simulink model "sensorExpoler_lab_Encoder"  (R2026a)
settings: Solver=FixedStepAuto  StopTime=inf  FixedStep=0.001
libraries: simulink x2, amg_usbconverter_n_connect_lib x2, dspfdesign x1
settings Model: Creator=pboon  LastModifiedBy=User

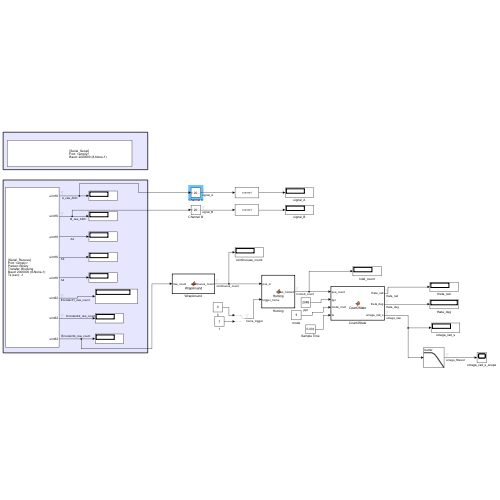
[thumbnail: Simulink's stored preview of the top-level diagram]
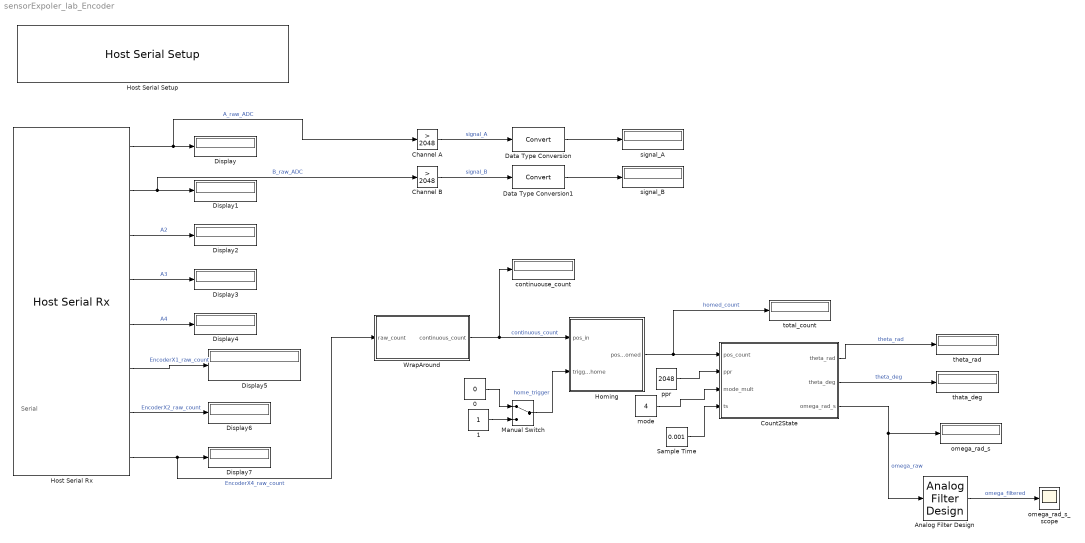
== system sensorExpoler_lab_Encoder ==
  note: Serial
  0 : Constant  Value=0
  1 : Constant
  Analog Filter Design : dspfdesign/Analog Filter Design  method=Butterworth  filttype=Lowpass  N=2  Wlo=30  Whi=80  Rp=2  Rs=40
  Channel A : simulink/Logic and Bit Operations/Compare To Constant  relop=>  const=2048  OutDataTypeStr=boolean
  Channel B : simulink/Logic and Bit Operations/Compare To Constant  relop=>  const=2048  OutDataTypeStr=boolean
  Count2State : MATLAB Function  TreatAsAtomicUnit=on
  Data Type Conversion : DataTypeConversion  SaturateOnIntegerOverflow=off  RndMeth=Floor
  Data Type Conversion1 : DataTypeConversion  SaturateOnIntegerOverflow=off  RndMeth=Floor
  Display{,1..7} (8 alike) : Display
  Homing : MATLAB Function  TreatAsAtomicUnit=on
  Host Serial Rx : amg_usbconverter_n_connect_lib/Host Serial Rx  conf=rx  port=<auto>  baudrate=2000000  databits=8  parity=None  stopbit=1  flowcontrol=None  transfer=Blocking  timeout=5  packetmode=Binary  enableinitialvalues=off  initialvalues=[]  binheader='25'  binterminator='4E 4E'  porttype_double=0  porttype_single=0  porttype_int8=0  porttype_uint8=0  porttype_int16=0  porttype_uint16=5  porttype_int32=0  porttype_uint32=3  asciiformat='%d,%f'  rx_asciiterminator="CRLF (0x0D 0x0A - \"\\r\\n\")"  tx_asciiterminator="CRLF (0x0D 0x0A - \"\\r\\n\")"  sampletime=0.001  enablecustomportlabel=off  cinputportlabel=0  coutputportlabel=A  portpinstr=0  blockid=HostSerialRx  inputporttype=[]  inputportwidth=[]  inputportlabel={}  outputporttype=[5 5 5 5 5 7 7 7]  outputportwidth=[1 1 1 1 1 1 1 1]  outputportlabel={'uint16','uint16','uint16','uint16','uint16','uint32','uint32','uint32'}  compat=0  optionstring=[]  autoport='<empty>'
  Host Serial Setup : amg_usbconverter_n_connect_lib/Host Serial Setup  conf=setup  port=<auto>  baudrate=2000000  databits=8  parity=None  stopbit=1  flowcontrol=None  transfer=Blocking  timeout=2  packetmode=Binary  initialvalues=[]  binheader='7E 7E'  binterminator='03 03'  porttype_double=0  porttype_single=1  porttype_int8=0  porttype_uint8=0  porttype_int16=0  porttype_uint16=0  porttype_int32=0  porttype_uint32=2  asciiformat='%d %u %x'  rx_asciiterminator="CRLF (0x0D 0x0A - \"\\r\\n\")"  tx_asciiterminator="CRLF (0x0D 0x0A - \"\\r\\n\")"  sampletime=-1  enablecustomportlabel=off  cinputportlabel=0  coutputportlabel=A  portpinstr=0  blockid=HostSerialSetup  inputporttype=[]  inputportwidth=[]  inputportlabel={}  outputporttype=[]  outputportwidth=[]  outputportlabel={}  compat=0  optionstring=[]  autoport='<empty>'
  Manual Switch : ManualSwitch
  Sample Time : Constant  Value=0.001
  WrapAround : MATLAB Function  TreatAsAtomicUnit=on
  continuouse_count : Display
  mode : Constant  Value=4
  omega_rad_s : Display
  omega_rad_s_scope : Scope
      settings: ActiveDisplayYMinimum=-168.77272661453941  ActiveDisplayYMaximum=441.86946444637664
  ppr : Constant  Value=2048
  signal_A : Display
  signal_B : Display
  thata_deg : Display
  theta_rad : Display
  total_count : Display
  wires:
  Host Serial Rx/1 -> Channel A/1, Display/1  "A_raw_ADC"
  Host Serial Rx/2 -> Channel B/1, Display1/1  "B_raw_ADC"
  Host Serial Rx/3 -> Display2/1  "A2"
  Host Serial Rx/4 -> Display3/1  "A3"
  Host Serial Rx/7 -> Display6/1  "EncoderX2_raw_count"
  Host Serial Rx/8 -> WrapAround/1(raw_count), Display7/1  "EncoderX4_raw_count"
  Manual Switch/1 -> Homing/2(trigger_home)  "home_trigger"
  ppr/1 -> Count2State/2(ppr)
  mode/1 -> Count2State/3(mode_mult)
  Sample Time/1 -> Count2State/4(ts)
  WrapAround/1(continuous_count) -> continuouse_count/1, Homing/1(pos_in)  "continuous_count"
  1/1 -> Manual Switch/2
  0/1 -> Manual Switch/1
  Count2State/1(theta_rad) -> theta_rad/1  "theta_rad"
  Count2State/2(theta_deg) -> thata_deg/1  "theta_deg"
  Count2State/3(omega_rad_s) -> Analog Filter Design/1, omega_rad_s/1  "omega_raw"
  Host Serial Rx/5 -> Display4/1  "A4"
  Host Serial Rx/6 -> Display5/1  "EncoderX1_raw_count"
  Homing/1(pos_homed) -> total_count/1, Count2State/1(pos_count)  "homed_count"
  Analog Filter Design/1 -> omega_rad_s_scope/1  "omega_filtered"
  Channel A/1 -> Data Type Conversion/1  "signal_A"
  Channel B/1 -> Data Type Conversion1/1  "signal_B"
  Data Type Conversion/1 -> signal_A/1
  Data Type Conversion1/1 -> signal_B/1

== matlab function sensorExpoler_lab_Encoder/Count2State ==
  data: pos_count input; theta_rad output; ppr input; mode_mult input; ts input; theta_deg output; omega_rad_s output
function [theta_rad, theta_deg, omega_rad_s] = Count2State(pos_count, ppr, mode_mult, ts)
    counts_per_rev = double(ppr) * double(mode_mult);
    
    % คำนวณตำแหน่งเชิงมุม
    theta_rad = (double(pos_count) / counts_per_rev) * (2 * pi);
    theta_deg = (double(pos_count) / counts_per_rev) * 360.0;
    
    % คำนวณความเร็วเชิงมุม
    persistent last_theta;
    if isempty(last_theta)
        last_theta = theta_rad;
    end
    
    delta_theta = theta_rad - last_theta;
    omega_rad_s = delta_theta / ts;
    last_theta = theta_rad;
end

== matlab function sensorExpoler_lab_Encoder/Homing ==
  data: pos_in input; pos_homed output; trigger_home input
function pos_homed = Homing(pos_in, trigger_home)
    persistent home_offset;
    
    if isempty(home_offset)
        home_offset = 0;
    end
    
    if trigger_home > 0
        home_offset = pos_in;
    end
    
    pos_homed = pos_in - home_offset;
end

== matlab function sensorExpoler_lab_Encoder/WrapAround ==
  data: raw_count input; continuous_count output
function continuous_count = WrapAround(raw_count)
 
    PERIOD = 65536; 
    HALF_PERIOD = PERIOD / 2; % 32768
    
    persistent last_raw;
    persistent total_pos;
    
    if isempty(last_raw)
        last_raw = double(raw_count);
        total_pos = double(raw_count);
    end
    
    current_raw = double(raw_count);
    delta = current_raw - last_raw;
    
    % ดักจับ Overflow
    if delta < -HALF_PERIOD
        delta = delta + PERIOD;
    % ดักจับ Underflow
    elseif delta > HALF_PERIOD
        delta = delta - PERIOD;
    end
    
    total_pos = total_pos + delta;
    last_raw = current_raw;
    
    continuous_count = total_pos;
end
